simulink model "problem2alter"  (R2020b)
settings: Solver=VariableStepAuto  StartTime=0.0  StopTime=10.0  RelTol=1e-3
settings Model: Creator=Sourav Kumar  LastModifiedBy=Sourav Kumar
settings DataIOCC: ExternalInput=[t, sig]  LoadExternalInput=on  SaveFormat=Array

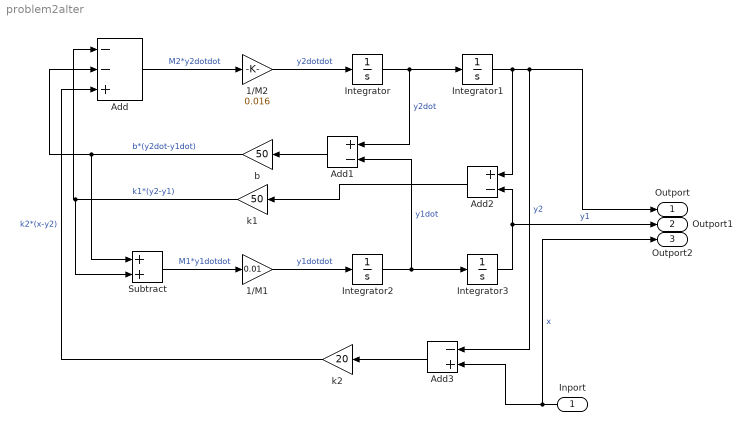
== system problem2alter ==
  Inport : Inport
  1/M1 : Gain  Gain=0.01
  1/M2 : Gain  Gain=0.016
  Add : Sum  Inputs=--+
  Add1 : Sum  Inputs=+-
  Add2 : Sum  Inputs=+-
  Add3 : Sum  Inputs=-+
  Integrator{,1..3} (4 alike) : Integrator
  Subtract : Sum
  b : Gain  Gain=50
  k1 : Gain  Gain=50
  k2 : Gain  Gain=20
  Outport : Outport
  Outport1 : Outport  Port=2
  Outport2 : Outport  Port=3
  wires:
  1/M1/1 -> Integrator2/1  "y1dotdot"
  Add/1 -> 1/M2/1  "M2*y2dotdot"
  Add3/1 -> k2/1
  Integrator/1 -> Add1/1, Integrator1/1  "y2dot"
  1/M2/1 -> Integrator/1  "y2dotdot"
  Integrator3/1 -> Outport1/1, Add2/2  "y1"
  Integrator2/1 -> Integrator3/1, Add1/2  "y1dot"
  k1/1 -> Subtract/2, Add/1  "k1*(y2-y1)"
  Inport/1 -> Outport2/1, Add3/2  "x"
  Add2/1 -> k1/1
  Add1/1 -> b/1
  k2/1 -> Add/3  "k2*(x-y2)"
  Subtract/1 -> 1/M1/1  "M1*y1dotdot"
  b/1 -> Subtract/1, Add/2  "b*(y2dot-y1dot)"
  Integrator1/1 -> Outport/1, Add3/1, Add2/1  "y2"
